simulink model "pendulum"  (R2023a)
settings: Solver=ode8  StartTime=0.0  StopTime=10.0  FixedStep=0.005  RelTol=1e-3
undefined symbols (not defined in the file): K
settings Model: Creator=rout3  LastModifiedBy=rout3

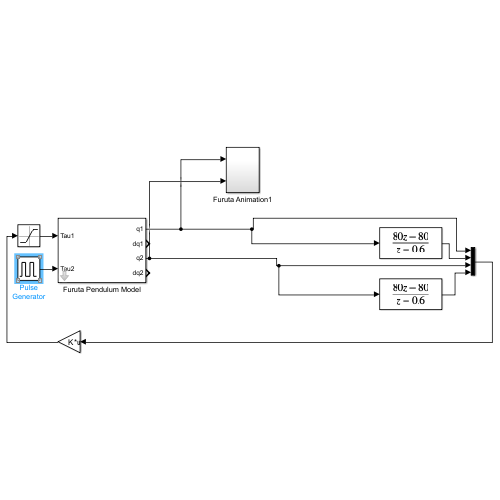
[thumbnail: Simulink's stored preview of the top-level diagram]
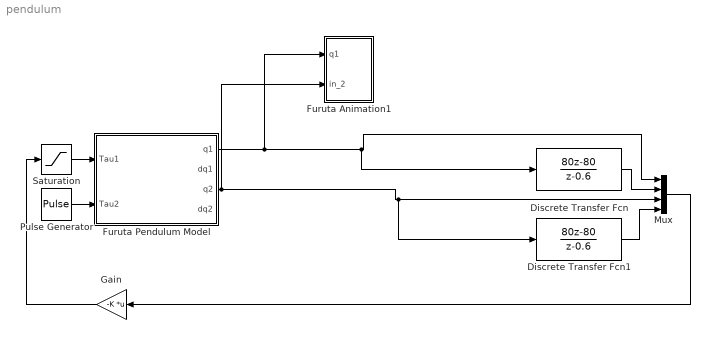
== system pendulum ==
  Discrete Transfer Fcn : DiscreteTransferFcn  Numerator=[80 -80]  Denominator=[1 -0.6]  SampleTime=0.005
  Discrete Transfer Fcn1 : DiscreteTransferFcn  Numerator=[80 -80]  Denominator=[1 -0.6]  SampleTime=0.005
  Furuta Animation1 : Subsystem
  Furuta Pendulum Model : Subsystem  mask{par=[0.0395, 0.0327, 0.0370, 0.0270, 0.3974], g=9.804, init=[0 0 0.1 0]}
      mask prompts: par "parameters"; g "acceleration of gravity"; init "Initial Conditions"
  Gain : Gain  Gain=-K  Multiplication=Matrix(K*u)
  Mux : Mux
  Pulse Generator : DiscretePulseGenerator  PulseType=Time based  Amplitude=2  Period=4  PulseWidth=4  PhaseDelay=4
  Saturation : Saturate  UpperLimit=10  LowerLimit=-10
  wires:
  Furuta Pendulum Model/1(q1) -> Furuta Animation1/1(q1), Discrete Transfer Fcn/1, Mux/1
  Discrete Transfer Fcn/1 -> Mux/2
  Discrete Transfer Fcn1/1 -> Mux/4
  Mux/1 -> Gain/1
  Saturation/1 -> Furuta Pendulum Model/1(Tau1)
  Gain/1 -> Saturation/1
  Furuta Pendulum Model/3(q2) -> Furuta Animation1/2(in_2), Discrete Transfer Fcn1/1, Mux/3
  Pulse Generator/1 -> Furuta Pendulum Model/2(Tau2)

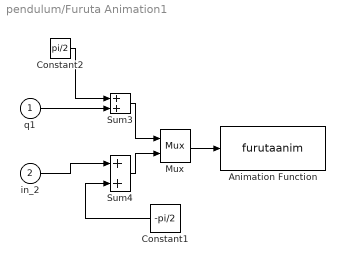
== system pendulum/Furuta Animation1 ==
  q1 : Inport
  in_2 : Inport  Port=2
  Animation Function : S-Function  FunctionName=furutaanim  Parameters=0.05  SFunctionDeploymentMode=off  EnableBusSupport=off
      settings: DeleteFcn=if ~isempty(findobj('type','figure','name','dblpend1 Animation'));close('dblpend1 Animation'); end;
  Constant1 : Constant  Value=-pi/2
  Constant2 : Constant  Value=pi/2
  Mux : Mux  Inputs=2
  Sum3 : Sum  InputSameDT=on  SaturateOnIntegerOverflow=on  OutDataTypeStr=Inherit: Same as first input
  Sum4 : Sum  InputSameDT=on  SaturateOnIntegerOverflow=on  OutDataTypeStr=Inherit: Same as first input
  wires:
  q1/1 -> Sum3/2
  Constant2/1 -> Sum3/1
  Sum3/1 -> Mux/1
  Sum4/1 -> Mux/2
  Mux/1 -> Animation Function/1
  Constant1/1 -> Sum4/2
  in_2/1 -> Sum4/1

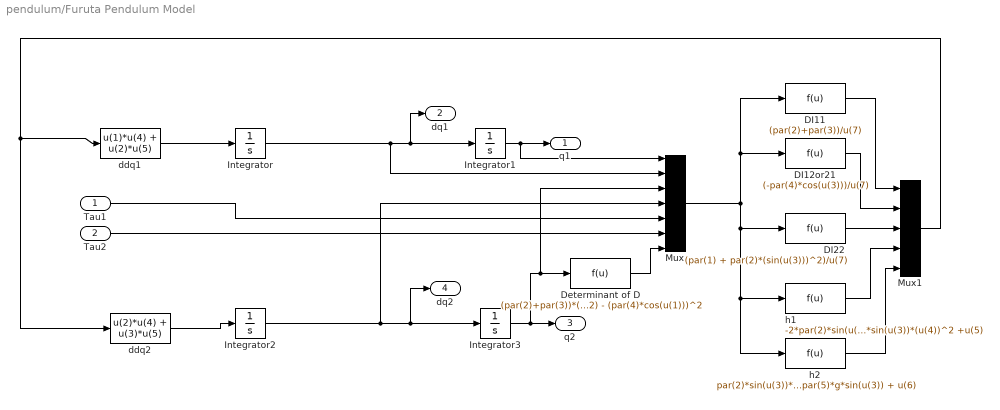
== system pendulum/Furuta Pendulum Model ==
  Tau1 : Inport
  Tau2 : Inport  Port=2
  DI11 : Fcn  Expr=(par(2)+par(3))/u(7)
  DI12or21 : Fcn  Expr=(-par(4)*cos(u(3)))/u(7)
  DI22 : Fcn  Expr=(par(1) + par(2)*(sin(u(3)))^2)/u(7)
  Determinant of D : Fcn  Expr=(par(2)+par(3))*(par(1) + par(2)*(sin(u(1)))^2) - (par(4)*cos(u(1)))^2
  Integrator : Integrator  InitialCondition=init(2)
  Integrator1 : Integrator  InitialCondition=init(1)
  Integrator2 : Integrator  InitialCondition=init(4)
  Integrator3 : Integrator  InitialCondition=init(3)
  Mux : Mux  Inputs=7
  Mux1 : Mux  Inputs=5
  ddq1 : Fcn  Expr=u(1)*u(4) + u(2)*u(5)
  ddq2 : Fcn  Expr=u(2)*u(4) + u(3)*u(5)
  h1 : Fcn  Expr=-2*par(2)*sin(u(3))*cos(u(3))*u(2)*u(4)+par(4)*sin(u(3))*(u(4))^2 +u(5)
  h2 : Fcn  Expr=par(2)*sin(u(3))*cos(u(3))*(u(2))^2 + par(5)*g*sin(u(3)) + u(6)
  q1 : Outport
  dq1 : Outport  Port=2
  q2 : Outport  Port=3
  dq2 : Outport  Port=4
  wires:
  Integrator3/1 -> q2/1, Determinant of D/1, Mux/3
  Integrator1/1 -> q1/1, Mux/1
  Integrator/1 -> Integrator1/1, dq1/1, Mux/2
  Integrator2/1 -> Integrator3/1, dq2/1, Mux/4
  Tau2/1 -> Mux/6
  Tau1/1 -> Mux/5
  Mux/1 -> h2/1, h1/1, DI22/1, DI11/1, DI12or21/1
  DI22/1 -> Mux1/3
  h1/1 -> Mux1/4
  h2/1 -> Mux1/5
  DI12or21/1 -> Mux1/2
  DI11/1 -> Mux1/1
  Mux1/1 -> ddq2/1, ddq1/1
  ddq2/1 -> Integrator2/1
  ddq1/1 -> Integrator/1
  Determinant of D/1 -> Mux/7
